simulink model "HILClimbers_LED_Rear_Light_Module_V6"  (R2021a)
settings: Solver=VariableStepAuto  StartTime=0.0  StopTime=400  RelTol=1e-3
model workspace (MAT data in the model file):
  brake = 0
undefined symbols (not defined in the file): sigbuilder_block
settings Model: PauseTimes=60  Creator=Sai229  LastModifiedBy=Sai229

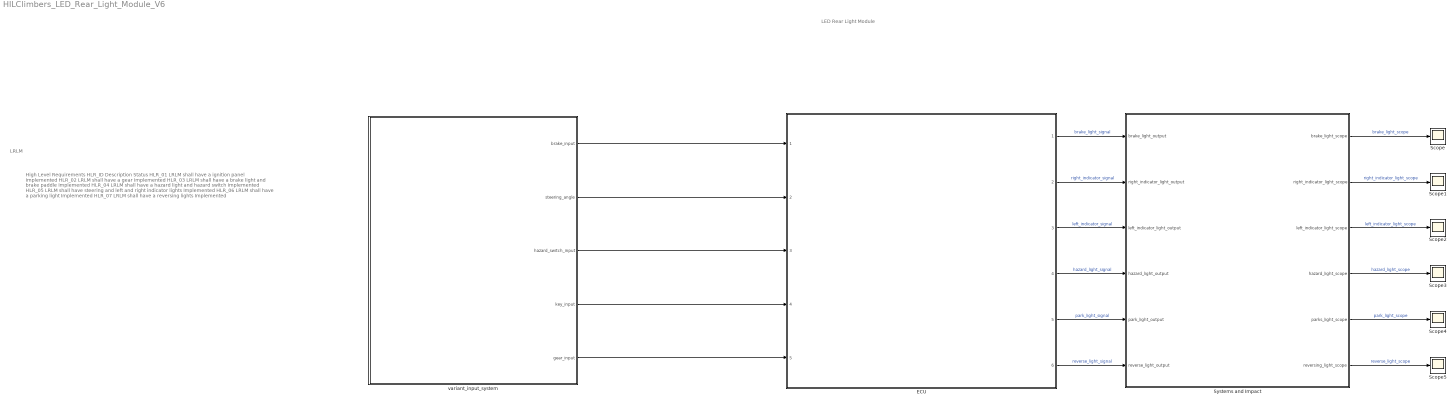
== system HILClimbers_LED_Rear_Light_Module_V6 ==
  note: LRLM
  note: High Level Requirements
      |
      | HLR_ID
      | Description
      | Status
      |
      | HLR_01
      | LRLM shall have a ignition panel
      | Implemented
      |
      | HLR_02
      | LRLM shall have a gear
      | Implemented
      |
      | HLR_03
      | LRLM shall have a brake light and brake paddle
      | Implemented
      |
      | HLR_04
      | LRLM shall have a hazard light and hazard switch
      | Implemented
      |
      | HLR_05
      | LRLM shall have steering and left and right indicator lights
      | Implemented
      |
      | HLR_06
      | LRLM shall have a parking light
      | Implemented
      |
      | HLR_07
      | LRLM shall have a reversing lights
      | Implemented
  note: LED Rear Light Module
  ECU : Subsystem  ReferencedSubsystem=LRLM_ECU
  Scope{,1..5} (6 alike) : Scope
  Systems and Impact : Subsystem
  variant_input_system : Subsystem  InitFcn=|  Variant=on
      | manual_test=Simulink.Variant("test_mode==0");
      | automated_test=Simulink.Variant("test_mode==1");
  wires:
  ECU/1 -> Systems and Impact/1(brake_light_output)  "brake_light_signal"
  ECU/2 -> Systems and Impact/2(right_indicator_light_output)  "right_indicator_signal"
  ECU/3 -> Systems and Impact/3(left_indicator_light_output)  "left_indicator_signal"
  ECU/4 -> Systems and Impact/4(hazard_light_output)  "hazard_light_signal"
  ECU/5 -> Systems and Impact/5(park_light_output)  "park_light_signal"
  ECU/6 -> Systems and Impact/6(reverse_light_output)  "reverse_light_signal"
  Systems and Impact/1(brake_light_scope) -> Scope/1  "brake_light_scope"
  Systems and Impact/3(left_indicator_light_scope) -> Scope2/1  "left_indicator_light_scope"
  Systems and Impact/4(hazard_light_scope) -> Scope3/1  "hazard_light_scope"
  Systems and Impact/5(parks_light_scope) -> Scope4/1  "park_light_scope"
  Systems and Impact/6(reversing_light_scope) -> Scope5/1  "reverse_light_scope"
  Systems and Impact/2(right_indicator_light_scope) -> Scope1/1  "right_indicator_light_scope"
  variant_input_system/1(brake_input) -> ECU/1
  variant_input_system/2(steering_angle) -> ECU/2
  variant_input_system/3(hazard_switch_input) -> ECU/3
  variant_input_system/4(key_input) -> ECU/4
  variant_input_system/5(gear_input) -> ECU/5

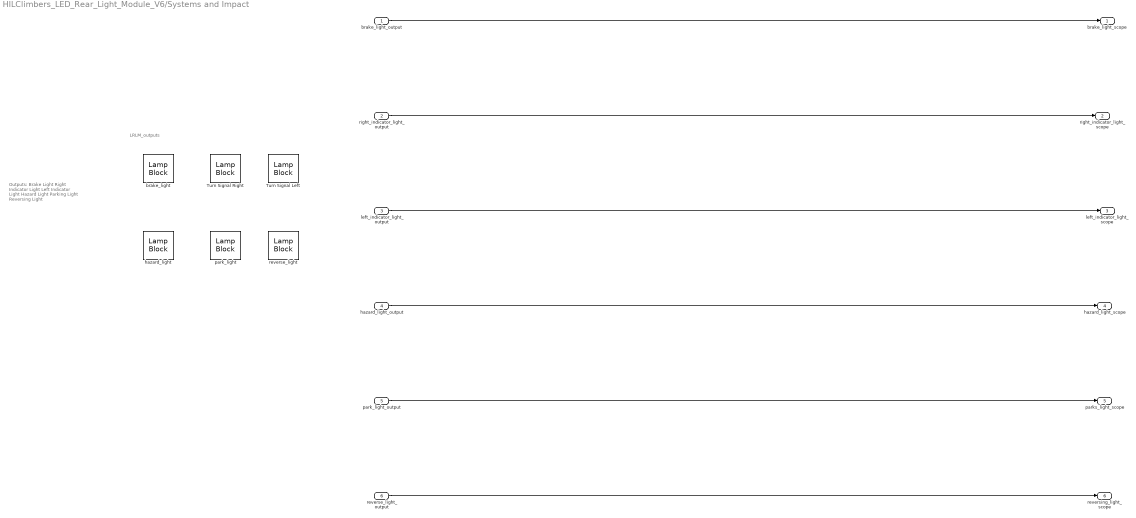
== system HILClimbers_LED_Rear_Light_Module_V6/Systems and Impact ==
  note: Outputs:
      | Brake Light
      | Right Indicator Light
      | Left Indicator Light
      | Hazard Light
      | Parking Light
      | Reversing Light
  note: LRLM_outputs
  brake_light_output : Inport
  right_indicator_light_output : Inport  Port=2
  left_indicator_light_output : Inport  Port=3
  hazard_light_output : Inport  Port=4
  park_light_output : Inport  Port=5
  reverse_light_output : Inport  Port=6
  Turn Signal Left : LampBlock  LabelPosition=Hide  Icon=TurnSignalLeft
  Turn Signal Right : LampBlock  LabelPosition=Hide  Icon=TurnSignalRight
  brake_light : LampBlock  LabelPosition=Hide  Icon=LightingSwitch
  hazard_light : LampBlock  LabelPosition=Hide  Icon=Hazards
  park_light : LampBlock  Icon=ParkingAssistance
  reverse_light : LampBlock  Icon=RearFogLight
  brake_light_scope : Outport
  right_indicator_light_scope : Outport  Port=2
  left_indicator_light_scope : Outport  Port=3
  hazard_light_scope : Outport  Port=4
  parks_light_scope : Outport  Port=5
  reversing_light_scope : Outport  Port=6
  wires:
  hazard_light_output/1 -> hazard_light_scope/1
  reverse_light_output/1 -> reversing_light_scope/1
  park_light_output/1 -> parks_light_scope/1
  left_indicator_light_output/1 -> left_indicator_light_scope/1
  right_indicator_light_output/1 -> right_indicator_light_scope/1
  brake_light_output/1 -> brake_light_scope/1

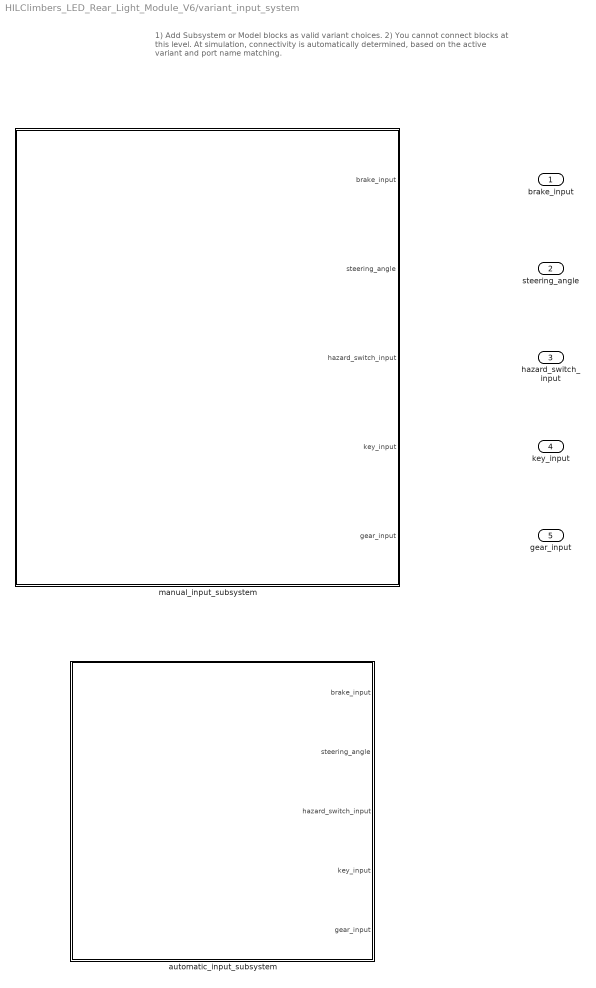
== system HILClimbers_LED_Rear_Light_Module_V6/variant_input_system ==
  note: 1) Add Subsystem or Model blocks as valid variant choices.
      | 2) You cannot connect blocks at this level. At simulation, connectivity is automatically
      | determined, based on the active variant and port name matching.
  automatic_input_subsystem : Subsystem  VariantControl=automated_test
  manual_input_subsystem : Subsystem  VariantControl=manual_test
  brake_input : Outport
  steering_angle : Outport  Port=2
  hazard_switch_input : Outport  Port=3
  key_input : Outport  Port=4
  gear_input : Outport  Port=5

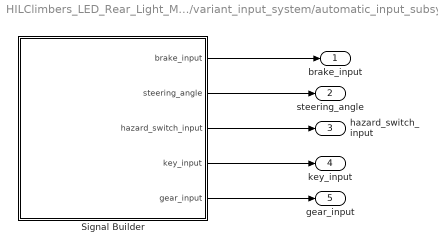
== system HILClimbers_LED_Rear_Light_Module_V6/variant_input_system/automatic_input_subsystem ==
  Signal Builder : Subsystem  Tag=STV Subsys  LoadFcn=sigbuilder_block('load');  StartFcn=sigbuilder_block('start');  StopFcn=sigbuilder_block('stop');  ClipboardFcn=sigbuilder_block('clipboard');  mask(Sigbuilder block){tuvar=[0:10]}
      mask help: Simulink:masks:SigbuilderBlock_MD
      mask init:
      | if ~strcmp(get_param(bdroot(gcbh),'SimulationStatus'),'stopped') tuvar = sigbuilder_block('maskInit'); end
      settings: CopyFcn=sigbuilder_block('copy');  DeleteFcn=sigbuilder_block('delete');  ModelCloseFcn=sigbuilder_block('modelClose');  PreSaveFcn=sigbuilder_block('preSave');  PauseFcn=sigbuilder_block('pause');  ContinueFcn=sigbuilder_block('continue');  NameChangeFcn=sigbuilder_block('namechange');  OpenFcn=sigbuilder_block('open',[5.4 30 1141.2 522.6 ]);  CloseFcn=sigbuilder_block('close');
      mask Display: plot(0, 0, 100, 100,[2, 2, 32, 32, 2], [68, 8, 8, 68, 68],[32, 2], [38, 38], [32, 19, 2],[53, 60, 44], [32, 17, 17, 2],[16, 16, 31, 31]);txt = getActiveGroup(gcbh);text(2, 100, txt,'verticalAlignment', 'top');
  brake_input : Outport
  steering_angle : Outport  Port=2
  hazard_switch_input : Outport  Port=3
  key_input : Outport  Port=4
  gear_input : Outport  Port=5
  wires:
  Signal Builder/1(brake_input) -> brake_input/1
  Signal Builder/5(gear_input) -> gear_input/1
  Signal Builder/3(hazard_switch_input) -> hazard_switch_input/1
  Signal Builder/2(steering_angle) -> steering_angle/1
  Signal Builder/4(key_input) -> key_input/1

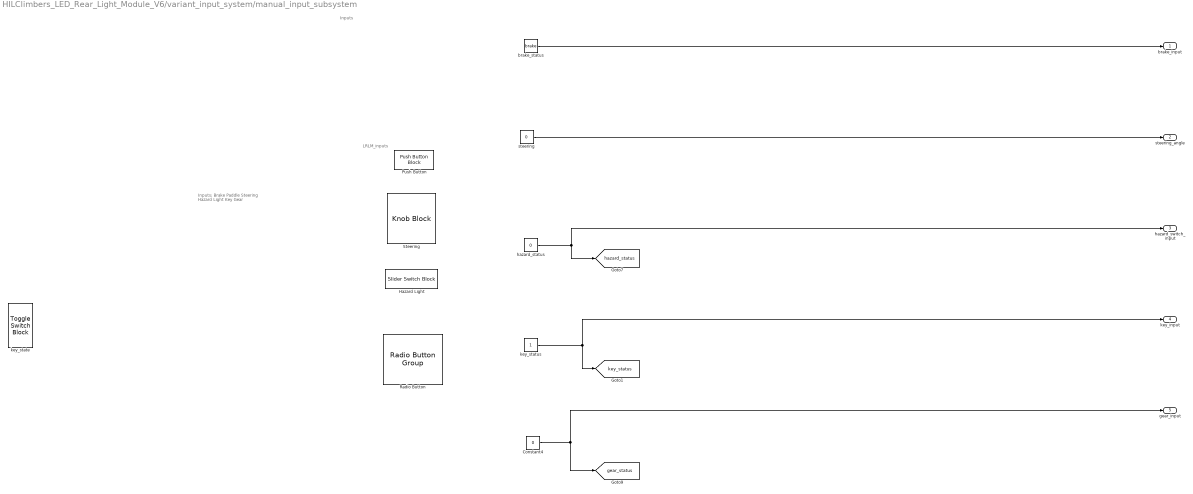
== system HILClimbers_LED_Rear_Light_Module_V6/variant_input_system/manual_input_subsystem ==
  note: Inputs
  note: LRLM_inputs
  note: Inputs:
      | Brake Paddle
      | Steering
      | Hazard Light
      | Key
      | Gear
  Constant4 : Constant  Value=0
  Hazard Light : SliderSwitchBlock  LabelPosition=Hide
      settings: Values={{'Off', 'On'}, [0 1]}
  Push Button : PushButtonBlock  ButtonText=Brake
  Radio Button : RadioButtonGroup  LabelPosition=Hide  SelectedLabel=Neutral  ButtonGroupName=Gear
      settings: Values={{'Neutral', 'Drive', 'Park', 'Reverse'}, [0 1 2 3]}
  Steering : KnobBlock  LabelPosition=Hide  ScaleMin=-90  ScaleMax=90  TickInterval=45
  brake_status : Constant  Value=brake
  hazard_status : Constant  Value=0
  key_state : ToggleSwitchBlock  LabelPosition=Bottom
      settings: Values={{'Off', 'On'}, [0 1]}
  key_status : Constant
  steering : Constant  Value=0
  brake_input : Outport
  steering_angle : Outport  Port=2
  hazard_switch_input : Outport  Port=3
  key_input : Outport  Port=4
  gear_input : Outport  Port=5
  tag scope: gear_status=global, hazard_status=global, key_status=global
  wires:
  brake_status/1 -> brake_input/1
  Constant4/1 -> [gear_status], gear_input/1
  steering/1 -> steering_angle/1
  key_status/1 -> [key_status], key_input/1
  hazard_status/1 -> hazard_switch_input/1, [hazard_status]

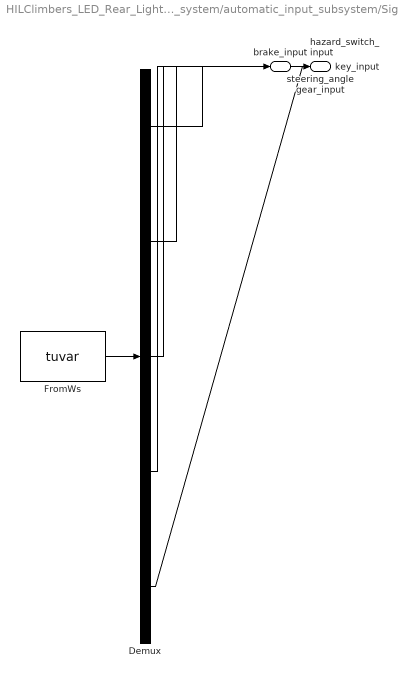
== system HILClimbers_LED_Rear_Light_Module_V6/variant_input_system/automatic_input_subsystem/Signal Builder ==
  Demux : Demux  Tag=STV Demux  Outputs=5
      settings: DisplayOption=none
  FromWs : FromWorkspace  Tag=STV FromWs  VariableName=tuvar
      SigBuilderData=|
      | common.afterFinalStr = 'Extrapolate'
      | common.sampleTime = 0
      | dataSet.timeRange = [0 160]
      | dataSet.name = 'inputs'
      | sbobj.Name = 'Signal Builder'
      | sbobj.Groups.Name = 'inputs'
      | sbobj.Groups.Signals(1).Name = 'brake_input'
      | sbobj.Groups.Signals(1).XData = [0 1 2 3 4 5 6 7 8 9 10 11 12 13 14 15 16 17 18 19 20 21 22 23 24 25 26 27 28 29 30 31 32 33 34 35 36 37 38 39 40 41 42 43 44 45 46 47 48 49 50 51 52 53 54 55 56 57 58 59 60 61 62 63 64 65 66 67 68 69 70 71 72 73 74 75 76 77 78 79 80 80 81 82 83 84 85 86 87 88 89 90 91 92 93 94 95 96 97 98 99 100 101 102 103 104 105 106 107 108 109 110 111 112 113 114 115 116 117 118 119 120 121 122 123 124 125 126 127 128 129 130 131 132 133 134 135 136 137 138 139 140 141 142 143 144 145 146 147 148 149 150 151 152 153 154 155 156 157 158 159 160]
      | sbobj.Groups.Signals(1).YData = [0 0 0 0 0 0 0 0 0 0 0 0 0 0 0 0 0 0 0 0 0 0 0 0 0 0 0 0 0 0 0 0 0 0 0 0 0 0 0 0 0 0 0 0 0 0 0 0 0 0 0 0 0 0 0 0 0 0 0 0 0 0 0 0 0 0 0 0 0 0 0 0 0 0 0 0 0 0 0 0 0 1 1 1 1 1 1 1 1 1 1 1 1 1 1 1 1 1 1 1 1 1 1 1 1 1 1 1 1 1 1 1 1 1 1 1 1 1 1 1 1 1 1 1 1 1 1 1 1 1 1 1 1 1 1 1 1 1 1 1 1 1 1 1 1 1 1 1 1 1 1 1 1 1 1 1 1 1 1 1 1 1]
      | sbobj.Groups.Signals(2).Name = 'steering_angle'
      | sbobj.Groups.Signals(2).XData = [0 1 2 3 4 5 6 7 8 9 10 11 12 13 14 15 16 16 17 18 19 20 21 22 23 24 25 26 27 28 29 30 31 32 32 33 34 35 36 37 38 39 40 41 42 43 44 45 46 47 48 48 49 50 51 52 53 54 55 56 57 58 59 60 61 62 63 64 64 65 66 67 68 69 70 71 72 73 74 75 76 77 78 79 80 80 81 82 83 84 85 86 87 88 89 90 91 92 93 94 95 96 96 97 98 99 100 101 102 103 104 105 106 107 108 109 110 111 112 112 113 114 115 116 117 118 119 120 121 122 123 124 125 126 127 128 128 129 130 131 132 133 134 135 136 137 138 139 140 141 142 143 144 144 145 146 147 148 149 150 151 152 153 154 155 156 157 158 159 160]
      | sbobj.Groups.Signals(2).YData = [-90 -90 -90 -90 -90 -90 -90 -90 -90 -90 -90 -90 -90 -90 -90 -90 -90 -45 -45 -45 -45 -45 -45 -45 -45 -45 -45 -45 -45 -45 -45 -45 -45 -45 0 0 0 0 0 0 0 0 0 0 0 0 0 0 0 0 0 45 45 45 45 45 45 45 45 45 45 45 45 45 45 45 45 45 90 90 90 90 90 90 90 90 90 90 90 90 90 90 90 90 90 -90 -90 -90 -90 -90 -90 -90 -90 -90 -90 -90 -90 -90 -90 -90 -90 -90 -45 -45 -45 -45 -45 -45 -45 -45 -45 -45 -45 -45 -45 -45 -45 -45 -45 0 0 0 0 0 0 0 0 0 0 0 0 0 0 0 0 0 45 45 45 45 45 45 45 45 45 45 45 45 45 45 45 45 45 90 90 90 90 90 90 90 90 90 90 90 90 90 90 90 90 90]
      | sbobj.Groups.Signals(3).Name = 'hazard_switch_input'
      | sbobj.Groups.Signals(3).XData = [0 1 2 3 4 5 6 7 8 8 9 10 11 12 13 14 15 16 16 17 18 19 20 21 22 23 24 24 25 26 27 28 29 30 31 32 32 33 34 35 36 37 38 39 40 40 41 42 43 44 45 46 47 48 48 49 50 51 52 53 54 55 56 56 57 58 59 60 61 62 63 64 64 65 66 67 68 69 70 71 72 72 73 74 75 76 77 78 79 80 80 81 82 83 84 85 86 87 88 88 89 90 91 92 93 94 95 96 96 97 98 99 100 101 102 103 104 104 105 106 107 108 109 110 111 112 112 113 114 115 116 117 118 119 120 120 121 122 123 124 125 126 127 128 128 129 130 131 132 133 134 135 136 136 137 138 139 140 141 142 143 144 144 145 146 147 148 149 150 151 152 152 153 154 155 156 157 158 159 160]
      | sbobj.Groups.Signals(3).YData = [0 0 0 0 0 0 0 0 0 1 1 1 1 1 1 1 1 1 0 0 0 0 0 0 0 0 0 1 1 1 1 1 1 1 1 1 0 0 0 0 0 0 0 0 0 1 1 1 1 1 1 1 1 1 0 0 0 0 0 0 0 0 0 1 1 1 1 1 1 1 1 1 0 0 0 0 0 0 0 0 0 1 1 1 1 1 1 1 1 1 0 0 0 0 0 0 0 0 0 1 1 1 1 1 1 1 1 1 0 0 0 0 0 0 0 0 0 1 1 1 1 1 1 1 1 1 0 0 0 0 0 0 0 0 0 1 1 1 1 1 1 1 1 1 0 0 0 0 0 0 0 0 0 1 1 1 1 1 1 1 1 1 0 0 0 0 0 0 0 0 0 1 1 1 1 1 1 1 1 1]
      | sbobj.Groups.Signals(4).Name = 'key_input'
      | sbobj.Groups.Signals(4).XData = [0 1 2 3 4 4 5 6 7 8 8 9 10 11 12 12 13 14 15 16 16 17 18 19 20 20 21 22 23 24 24 25 26 27 28 28 29 30 31 32 32 33 34 35 36 36 37 38 39 40 40 41 42 43 44 44 45 46 47 48 48 49 50 51 52 52 53 54 55 56 56 57 58 59 60 60 61 62 63 64 64 65 66 67 68 68 69 70 71 72 72 73 74 75 76 76 77 78 79 80 80 81 82 83 84 84 85 86 87 88 88 89 90 91 92 92 93 94 95 96 96 97 98 99 100 100 101 102 103 104 104 105 106 107 108 108 109 110 111 112 112 113 114 115 116 116 117 118 119 120 120 121 122 123 124 124 125 126 127 128 128 129 130 131 132 132 133 134 135 136 136 137 138 139 140 140 141 142 143 144 144 145 146 147 148 148 149 150 151 152 152 153 154 155 156 156 157 158 159 160]
      | sbobj.Groups.Signals(4).YData = [0 0 0 0 0 1 1 1 1 1 0 0 0 0 0 1 1 1 1 1 0 0 0 0 0 1 1 1 1 1 0 0 0 0 0 1 1 1 1 1 0 0 0 0 0 1 1 1 1 1 0 0 0 0 0 1 1 1 1 1 0 0 0 0 0 1 1 1 1 1 0 0 0 0 0 1 1 1 1 1 0 0 0 0 0 1 1 1 1 1 0 0 0 0 0 1 1 1 1 1 0 0 0 0 0 1 1 1 1 1 0 0 0 0 0 1 1 1 1 1 0 0 0 0 0 1 1 1 1 1 0 0 0 0 0 1 1 1 1 1 0 0 0 0 0 1 1 1 1 1 0 0 0 0 0 1 1 1 1 1 0 0 0 0 0 1 1 1 1 1 0 0 0 0 0 1 1 1 1 1 0 0 0 0 0 1 1 1 1 1 0 0 0 0 0 1 1 1 1 1]
      | sbobj.Groups.Signals(5).Name = 'gear_input'
      | sbobj.Groups.Signals(5).XData = [0 1 1 2 2 3 3 4 4 5 5 6 6 7 7 8 8 9 9 10 10 11 11 12 12 13 13 14 14 15 15 16 16 17 17 18 18 19 19 20 20 21 21 22 22 23 23 24 24 25 25 26 26 27 27 28 28 29 29 30 30 31 31 32 32 33 33 34 34 35 35 36 36 37 37 38 38 39 39 40 40 41 41 42 42 43 43 44 44 45 45 46 46 47 47 48 48 49 49 50 50 51 51 52 52 53 53 54 54 55 55 56 56 57 57 58 58 59 59 60 60 61 61 62 62 63 63 64 64 65 65 66 66 67 67 68 68 69 69 70 70 71 71 72 72 73 73 74 74 75 75 76 76 77 77 78 78 79 79 80 80 81 81 82 82 83 83 84 84 85 85 86 86 87 87 88 88 89 89 90 90 91 91 92 92 93 93 94 94 95 95 96 96 97 97 98 98 99 99 100 100 101 101 102 102 103 103 104 104 105 105 106 106 107 107 108 108 109 109 110 110 111 111 112 112 113 113 114 114 115 115 116 116 117 117 118 118 119 119 120 120 121 121 122 122 123 123 124 124 125 125 126 126 127 127 128 128 129 129 130 130 131 131 132 132 133 133 134 134 135 135 136 136 137 137 138 138 139 139 140 140 141 141 142 142 143 143 144 144 145 145 146 146 147 147 148 148 149 149 150 150 151 151 152 152 153 153 154 154 155 155 156 156 157 157 158 158 159 159 160]
      | sbobj.Groups.Signals(5).YData = [0 0 1 1 2 2 3 3 0 0 1 1 2 2 3 3 0 0 1 1 2 2 3 3 0 0 1 1 2 2 3 3 0 0 1 1 2 2 3 3 0 0 1 1 2 2 3 3 0 0 1 1 2 2 3 3 0 0 1 1 2 2 3 3 0 0 1 1 2 2 3 3 0 0 1 1 2 2 3 3 0 0 1 1 2 2 3 3 0 0 1 1 2 2 3 3 0 0 1 1 2 2 3 3 0 0 1 1 2 2 3 3 0 0 1 1 2 2 3 3 0 0 1 1 2 2 3 3 0 0 1 1 2 2 3 3 0 0 1 1 2 2 3 3 0 0 1 1 2 2 3 3 0 0 1 1 2 2 3 3 0 0 1 1 2 2 3 3 0 0 1 1 2 2 3 3 0 0 1 1 2 2 3 3 0 0 1 1 2 2 3 3 0 0 1 1 2 2 3 3 0 0 1 1 2 2 3 3 0 0 1 1 2 2 3 3 0 0 1 1 2 2 3 3 0 0 1 1 2 2 3 3 0 0 1 1 2 2 3 3 0 0 1 1 2 2 3 3 0 0 1 1 2 2 3 3 0 0 1 1 2 2 3 3 0 0 1 1 2 2 3 3 0 0 1 1 2 2 3 3 0 0 1 1 2 2 3 3 0 0 1 1 2 2 3 3 0 0 1 1 2 2 3 3 0 0 1 1 2 2 3 3 0 0 1 1 2 2 3 3]
      | sbobj.Groups.TimeRange = [0 160]
  brake_input : Outport  Tag=STV Outport
  steering_angle : Outport  Tag=STV Outport  Port=2
  hazard_switch_input : Outport  Tag=STV Outport  Port=3
  key_input : Outport  Tag=STV Outport  Port=4
  gear_input : Outport  Tag=STV Outport  Port=5
  wires:
  Demux/1 -> brake_input/1
  FromWs/1 -> Demux/1
  Demux/2 -> steering_angle/1
  Demux/3 -> hazard_switch_input/1
  Demux/4 -> key_input/1
  Demux/5 -> gear_input/1
